simulink model "sldemo_mdlref_dsm_bot2"  (Simulink 7.6)
settings: Solver=FixedStepDiscrete  StartTime=0.0  StopTime=10.0  FixedStep=0.1  RelTol=1e-3
PreLoadFcn:
  | load sldemo_mdlref_dsm_data.mat
libraries: simulink x1
settings Model: Creator=The MathWorks Inc.  ExtModeAutoUpdateStatusClock=off
settings OptimizationCC: InlineParams=on  InitFltsAndDblsToZero=on
settings DebuggingCC: SaveWithParameterizedLinksMsg=none  MultiTaskCondExecSysMsg=none  SigSpecEnsureSampleTimeMsg=none  BusObjectLabelMismatch=error  RootOutportRequireBusObject=error  StrictBusMsg=ErrorOnBusTreatedAsVector
settings RTWCC: ProcessScript=grt_make_rtw_hook  IncludeERTFirstTime=on
settings CodeAppCC: MaxIdLength=100
settings GRTTargetCC: TargetFcnLib=ansi_tfl_tmw.mat

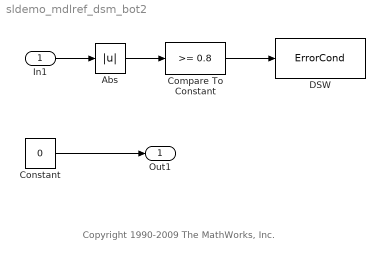
== system sldemo_mdlref_dsm_bot2 ==
  note: Copyright 1990-2009 The MathWorks, Inc.
  In1 : Inport  OutDataTypeStr=double  PortDimensions=1  SampleTime=0.1
  Abs : Abs
  Compare To Constant : simulink/Logic and Bit Operations/Compare To Constant  SystemSampleTime=-1  relop=>=  const=0.8  LogicOutDataTypeMode=boolean  ZeroCross=off
  Constant : Constant  Value=0
  DSW : DataStoreWrite  DataStoreName=ErrorCond  SampleTime=0.1
  Out1 : Outport
  wires:
  In1/1 -> Abs/1
  Compare To Constant/1 -> DSW/1
  Constant/1 -> Out1/1
  Abs/1 -> Compare To Constant/1
